simulink model "TST_LIB_FDI_ENCODEandDECODE"  (R2016b)
settings: Solver=VariableStepAuto  StartTime=0.0  StopTime=10.0  RelTol=1e-3
libraries: LIB_FDI x2
settings Model: Creator=alger  LastModifiedBy=alger

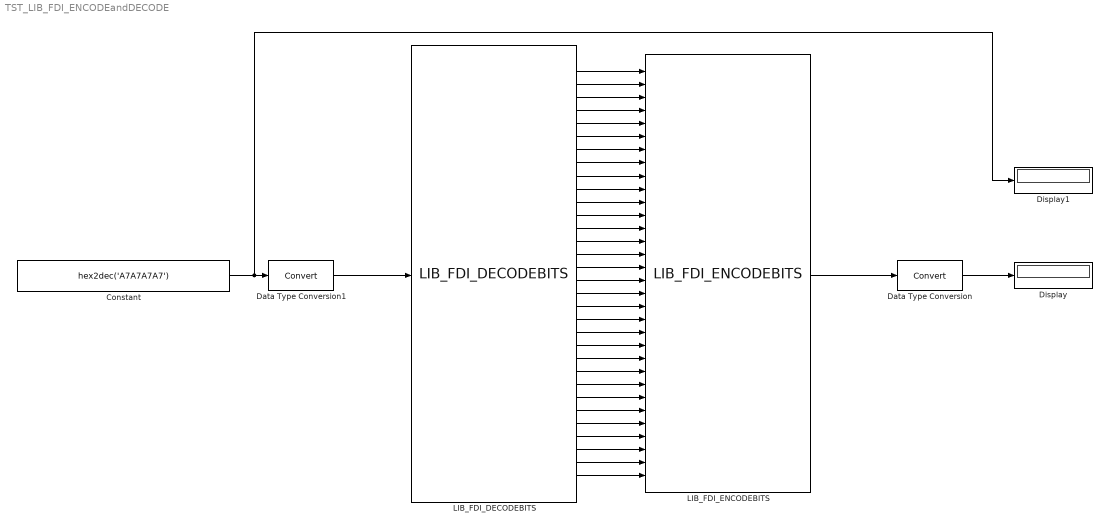
== system TST_LIB_FDI_ENCODEandDECODE ==
  Constant : Constant  Value=hex2dec('A7A7A7A7')
  Data Type Conversion : DataTypeConversion
  Data Type Conversion1 : DataTypeConversion
  Display : Display
  Display1 : Display
  LIB_FDI_DECODEBITS : LIB_FDI/LIB_FDI_DECODEBITS
  LIB_FDI_ENCODEBITS : LIB_FDI/LIB_FDI_ENCODEBITS
  wires:
  Constant/1 -> Display1/1, Data Type Conversion1/1
  LIB_FDI_ENCODEBITS/1 -> Data Type Conversion/1
  Data Type Conversion/1 -> Display/1
  Data Type Conversion1/1 -> LIB_FDI_DECODEBITS/1
  LIB_FDI_DECODEBITS/17 -> LIB_FDI_ENCODEBITS/17
  LIB_FDI_DECODEBITS/5 -> LIB_FDI_ENCODEBITS/5
  LIB_FDI_DECODEBITS/13 -> LIB_FDI_ENCODEBITS/13
  LIB_FDI_DECODEBITS/19 -> LIB_FDI_ENCODEBITS/19
  LIB_FDI_DECODEBITS/11 -> LIB_FDI_ENCODEBITS/11
  LIB_FDI_DECODEBITS/18 -> LIB_FDI_ENCODEBITS/18
  LIB_FDI_DECODEBITS/6 -> LIB_FDI_ENCODEBITS/6
  LIB_FDI_DECODEBITS/3 -> LIB_FDI_ENCODEBITS/3
  LIB_FDI_DECODEBITS/4 -> LIB_FDI_ENCODEBITS/4
  LIB_FDI_DECODEBITS/7 -> LIB_FDI_ENCODEBITS/7
  LIB_FDI_DECODEBITS/10 -> LIB_FDI_ENCODEBITS/10
  LIB_FDI_DECODEBITS/16 -> LIB_FDI_ENCODEBITS/16
  LIB_FDI_DECODEBITS/14 -> LIB_FDI_ENCODEBITS/14
  LIB_FDI_DECODEBITS/20 -> LIB_FDI_ENCODEBITS/20
  LIB_FDI_DECODEBITS/21 -> LIB_FDI_ENCODEBITS/21
  LIB_FDI_DECODEBITS/22 -> LIB_FDI_ENCODEBITS/22
  LIB_FDI_DECODEBITS/23 -> LIB_FDI_ENCODEBITS/23
  LIB_FDI_DECODEBITS/24 -> LIB_FDI_ENCODEBITS/24
  LIB_FDI_DECODEBITS/2 -> LIB_FDI_ENCODEBITS/2
  LIB_FDI_DECODEBITS/8 -> LIB_FDI_ENCODEBITS/8
  LIB_FDI_DECODEBITS/9 -> LIB_FDI_ENCODEBITS/9
  LIB_FDI_DECODEBITS/12 -> LIB_FDI_ENCODEBITS/12
  LIB_FDI_DECODEBITS/1 -> LIB_FDI_ENCODEBITS/1
  LIB_FDI_DECODEBITS/15 -> LIB_FDI_ENCODEBITS/15
  LIB_FDI_DECODEBITS/26 -> LIB_FDI_ENCODEBITS/26
  LIB_FDI_DECODEBITS/31 -> LIB_FDI_ENCODEBITS/31
  LIB_FDI_DECODEBITS/28 -> LIB_FDI_ENCODEBITS/28
  LIB_FDI_DECODEBITS/29 -> LIB_FDI_ENCODEBITS/29
  LIB_FDI_DECODEBITS/27 -> LIB_FDI_ENCODEBITS/27
  LIB_FDI_DECODEBITS/32 -> LIB_FDI_ENCODEBITS/32
  LIB_FDI_DECODEBITS/30 -> LIB_FDI_ENCODEBITS/30
  LIB_FDI_DECODEBITS/25 -> LIB_FDI_ENCODEBITS/25
